simulink model "pry_grasp_source"  (R2018b)
settings: Solver=FixedStepDiscrete  StartTime=0.0  StopTime=Inf  FixedStep=0.001  RelTol=1e-3
PostLoadFcn:
  | , if any(exist('dsrtsu_mdlpostloadfcn', 'file') ~= 0), dsrtsu_mdlpostloadfcn('Execute', bdroot); end,
undefined symbols (not defined in the file): b, Coulomb_friction, parallel_grasp, q1ini, q2ini, theta1, theta2, theta5, theta6, viscous_friction
libraries: simulink x26
(part 2 of 3)

== system pry_grasp_source/phase1/Enabled Subsystem7 ==
  enable : Inport
  angle_ref : Inport  Port=2
  angle : Inport  Port=3
  angle_vel : Inport  Port=4
  phase_time : Inport  Port=5
  end_time : Inport  Port=6
  Subsystem : Subsystem
  Triggered Subsystem : Subsystem  TreatAsAtomicUnit=on
  torque_out : Outport  OutputWhenDisabled=reset  InitialOutput=0
  wires:
  angle/1 -> Subsystem/6(current_angle), Triggered Subsystem/1(angle_In1)
  angle_ref/1 -> Triggered Subsystem/2(angle_ref_In2)
  end_time/1 -> Triggered Subsystem/3(end_time_In3)
  Triggered Subsystem/1(angle_Out1) -> Subsystem/1(initial_angle)
  Triggered Subsystem/2(angle_ref_Out2) -> Subsystem/2(end_angle)
  Triggered Subsystem/3(end_time_Out3) -> Subsystem/3(end_time)
  phase_time/1 -> Subsystem/4(time)
  angle_vel/1 -> Subsystem/5(angular_vel)
  Subsystem/1(torque_out) -> torque_out/1
  enable/1 -> Triggered Subsystem/Trigger, Subsystem/Enable

== system pry_grasp_source/phase1/Triggered Subsystem ==
  note: arm move downward
  In1 : Inport
  Trigger : TriggerPort  VariantControl=(inherit)
  Constant : Constant  Value=[0 1]
  Constant1 : Constant  Value=1.5
  Data Store Read : DataStoreRead  Priority=3  DataStoreName=phase_num
  Data Store Read4 : DataStoreRead  Priority=3  DataStoreName=UR_V
  Data Store Write : DataStoreWrite  DataStoreName=phase_num
  Data Store Write4 : DataStoreWrite  DataStoreName=UR_V
  Sum : Sum  Inputs=|++
  Sum1 : Sum  Inputs=|++
  Out1 : Outport
  wires:
  Data Store Read/1 -> Sum/1
  Sum/1 -> Data Store Write/1
  Constant/1 -> Sum/2
  Constant1/1 -> Sum1/2
  Sum1/1 -> Data Store Write4/1
  Data Store Read4/1 -> Sum1/1
  In1/1 -> Out1/1

== system pry_grasp_source/phase1/Triggered Subsystem1 ==
  In1 : Inport
  Trigger : TriggerPort  VariantControl=(inherit)
  Out1 : Outport  InitialOutput=0
  wires:
  In1/1 -> Out1/1

== system pry_grasp_source/phase1-1/Enabled Subsystem ==
  phase_start_time : Inport
  current_time : Inport  Port=2
  phase_end_time : Inport  Port=3
  Enable : EnablePort
  Relational Operator : RelationalOperator  OutDataTypeStr=boolean  RndMeth=Nearest
  Sum : Sum  Inputs=|-+
  phase_time : Outport  OutputWhenDisabled=reset  InitialOutput=0
  phase_end_signal : Outport  Port=2  OutputWhenDisabled=reset  InitialOutput=0
  wires:
  phase_start_time/1 -> Sum/1
  current_time/1 -> Sum/2
  Sum/1 -> phase_time/1, Relational Operator/1
  Relational Operator/1 -> phase_end_signal/1
  phase_end_time/1 -> Relational Operator/2

== system pry_grasp_source/phase1-1/Enabled Subsystem7 ==
  enable : Inport
  angle_ref : Inport  Port=2
  angle : Inport  Port=3
  angle_vel : Inport  Port=4
  Subsystem : Subsystem
  torque_out : Outport  OutputWhenDisabled=reset  InitialOutput=0
  wires:
  angle/1 -> Subsystem/3(current_angle)
  angle_ref/1 -> Subsystem/1(ref_angle)
  angle_vel/1 -> Subsystem/2(angular_vel)
  Subsystem/1(torque_out) -> torque_out/1
  enable/1 -> Subsystem/Enable

== system pry_grasp_source/phase1-1/Triggered Subsystem ==
  Trigger : TriggerPort  VariantControl=(inherit)
  Constant : Constant  Value=[0 1]
  Data Store Read : DataStoreRead  Priority=3  DataStoreName=phase_num
  Data Store Write : DataStoreWrite  DataStoreName=phase_num
  Sum : Sum  Inputs=|++
  wires:
  Data Store Read/1 -> Sum/1
  Sum/1 -> Data Store Write/1
  Constant/1 -> Sum/2

== system pry_grasp_source/phase1-1/Triggered Subsystem1 ==
  In1 : Inport
  Trigger : TriggerPort  VariantControl=(inherit)
  Out1 : Outport  InitialOutput=0
  wires:
  In1/1 -> Out1/1

== system pry_grasp_source/phase10/Enabled Subsystem1 ==
  In1 : Inport
  Enable : EnablePort
  Out1 : Outport  OutputWhenDisabled=reset  InitialOutput=0
  wires:
  In1/1 -> Out1/1

== system pry_grasp_source/phase10/Enabled Subsystem3 ==
  phase_start_time : Inport
  current_time : Inport  Port=2
  phase_end_time : Inport  Port=3
  Enable : EnablePort
  Relational Operator : RelationalOperator  OutDataTypeStr=boolean  RndMeth=Nearest
  Sum : Sum  Inputs=|-+
  phase_time : Outport  OutputWhenDisabled=reset  InitialOutput=0
  phase_end_signal : Outport  Port=2  OutputWhenDisabled=reset  InitialOutput=0
  wires:
  phase_start_time/1 -> Sum/1
  current_time/1 -> Sum/2
  Sum/1 -> phase_time/1, Relational Operator/1
  Relational Operator/1 -> phase_end_signal/1
  phase_end_time/1 -> Relational Operator/2

== system pry_grasp_source/phase10/Enabled Subsystem4 ==
  enable : Inport
  angle6 : Inport  Port=2
  angle5 : Inport  Port=3
  angular5_vel : Inport  Port=4
  angular6_vel : Inport  Port=5
  angle1 : Inport  Port=6
  angle2 : Inport  Port=7
  angular1_vel : Inport  Port=8
  angular2_vel : Inport  Port=9
  vel_x1 : Inport  Port=10
  Subsystem1 : Subsystem
  torque_out : Outport  OutputWhenDisabled=reset  InitialOutput=0
  wires:
  enable/1 -> Subsystem1/Enable
  Subsystem1/1(torque) -> torque_out/1
  angle5/1 -> Subsystem1/2(angle5)
  angle6/1 -> Subsystem1/1(angle6)
  angular5_vel/1 -> Subsystem1/3(angular5_vel)
  angular6_vel/1 -> Subsystem1/4(angular6_vel)
  angle1/1 -> Subsystem1/6(angle1)
  angle2/1 -> Subsystem1/5("angle2 ")
  angular1_vel/1 -> Subsystem1/7(angular1_vel)
  angular2_vel/1 -> Subsystem1/8(angular2_vel)
  vel_x1/1 -> Subsystem1/9(vel_x1)

== system pry_grasp_source/phase10/Triggered Subsystem1 ==
  Trigger : TriggerPort  VariantControl=(inherit)
  Constant : Constant  Value=[0 1]
  Data Store Read : DataStoreRead  Priority=3  DataStoreName=phase_num
  Data Store Write : DataStoreWrite  DataStoreName=phase_num
  Sum : Sum  Inputs=|++
  wires:
  Data Store Read/1 -> Sum/1
  Sum/1 -> Data Store Write/1
  Constant/1 -> Sum/2

== system pry_grasp_source/phase10/Triggered Subsystem4 ==
  Trigger : TriggerPort  VariantControl=(inherit)
  Constant : Constant  Value=[0 1]
  Data Store Read : DataStoreRead  Priority=3  DataStoreName=phase_num
  Data Store Write : DataStoreWrite  DataStoreName=phase_num
  Sum : Sum  Inputs=|++
  wires:
  Data Store Read/1 -> Sum/1
  Sum/1 -> Data Store Write/1
  Constant/1 -> Sum/2

== system pry_grasp_source/phase10/Triggered Subsystem5 ==
  In1 : Inport
  Trigger : TriggerPort  VariantControl=(inherit)
  Out1 : Outport  InitialOutput=0
  wires:
  In1/1 -> Out1/1

== system pry_grasp_source/phase11/Enabled Subsystem2 ==
  In1 : Inport
  Enable : EnablePort
  Out1 : Outport  OutputWhenDisabled=reset  InitialOutput=0
  wires:
  In1/1 -> Out1/1

== system pry_grasp_source/phase11/Enabled Subsystem3 ==
  phase_start_time : Inport
  current_time : Inport  Port=2
  phase_end_time : Inport  Port=3
  Enable : EnablePort
  Relational Operator : RelationalOperator  OutDataTypeStr=boolean  RndMeth=Nearest
  Sum : Sum  Inputs=|-+
  phase_time : Outport  OutputWhenDisabled=reset  InitialOutput=0
  phase_end_signal : Outport  Port=2  OutputWhenDisabled=reset  InitialOutput=0
  wires:
  phase_start_time/1 -> Sum/1
  current_time/1 -> Sum/2
  Sum/1 -> phase_time/1, Relational Operator/1
  Relational Operator/1 -> phase_end_signal/1
  phase_end_time/1 -> Relational Operator/2

== system pry_grasp_source/phase11/Enabled Subsystem4 ==
  enable : Inport
  angular5_in1 : Inport  Port=2
  angle2 : Inport  Port=3
  angle1 : Inport  Port=4
  angle6 : Inport  Port=5
  angle5 : Inport  Port=6
  Subsystem1 : Subsystem
  torque_out : Outport  OutputWhenDisabled=reset  InitialOutput=0
  wires:
  enable/1 -> Subsystem1/Enable
  Subsystem1/1(torque) -> torque_out/1
  angular5_in1/1 -> ?
  angle1/1 -> Subsystem1/2(angle1)
  angle2/1 -> Subsystem1/1("angle2 ")
  angle5/1 -> Subsystem1/4(angle5)
  angle6/1 -> Subsystem1/3(angle6)

== system pry_grasp_source/phase11/Triggered Subsystem3 ==
  In1 : Inport
  Trigger : TriggerPort  VariantControl=(inherit)
  Constant : Constant  Value=[0 1]
  Data Store Read : DataStoreRead  Priority=3  DataStoreName=phase_num
  Data Store Write : DataStoreWrite  DataStoreName=phase_num
  Sum : Sum  Inputs=|++
  Out1 : Outport
  wires:
  Data Store Read/1 -> Sum/1
  Sum/1 -> Data Store Write/1
  Constant/1 -> Sum/2
  In1/1 -> Out1/1

== system pry_grasp_source/phase11/Triggered Subsystem4 ==
  Trigger : TriggerPort  VariantControl=(inherit)
  Constant : Constant  Value=[0 1]
  Data Store Read : DataStoreRead  Priority=3  DataStoreName=phase_num
  Data Store Write : DataStoreWrite  DataStoreName=phase_num
  Sum : Sum  Inputs=|++
  wires:
  Data Store Read/1 -> Sum/1
  Sum/1 -> Data Store Write/1
  Constant/1 -> Sum/2

== system pry_grasp_source/phase11/Triggered Subsystem5 ==
  In1 : Inport
  Trigger : TriggerPort  VariantControl=(inherit)
  Out1 : Outport  InitialOutput=0
  wires:
  In1/1 -> Out1/1

== system pry_grasp_source/phase2/Enabled Subsystem ==
  phase_start_time : Inport
  current_time : Inport  Port=2
  phase_end_time : Inport  Port=3
  Enable : EnablePort
  Relational Operator : RelationalOperator  OutDataTypeStr=boolean  RndMeth=Nearest
  Sum : Sum  Inputs=|-+
  phase_time : Outport  OutputWhenDisabled=reset  InitialOutput=0
  phase_end_signal : Outport  Port=2  OutputWhenDisabled=reset  InitialOutput=0
  wires:
  phase_start_time/1 -> Sum/1
  current_time/1 -> Sum/2
  Sum/1 -> phase_time/1, Relational Operator/1
  Relational Operator/1 -> phase_end_signal/1
  phase_end_time/1 -> Relational Operator/2

== system pry_grasp_source/phase2/Enabled Subsystem7 ==
  enable : Inport
  ref_angle : Inport  Port=2
  angle : Inport  Port=3
  angle_vel : Inport  Port=4
  Subsystem : Subsystem
  torque_out : Outport  OutputWhenDisabled=reset  InitialOutput=0
  wires:
  angle/1 -> Subsystem/3(current_angle)
  angle_vel/1 -> Subsystem/2(angular_vel)
  Subsystem/1(torque_out) -> torque_out/1
  enable/1 -> Subsystem/Enable
  ref_angle/1 -> Subsystem/1(ref_angle)

== system pry_grasp_source/phase2/Triggered Subsystem ==
  In1 : Inport
  Trigger : TriggerPort  VariantControl=(inherit)
  Constant : Constant  Value=[0 1]
  Constant1 : Constant
  Data Store Read : DataStoreRead  Priority=3  DataStoreName=phase_num
  Data Store Read4 : DataStoreRead  Priority=3  DataStoreName=UR_V
  Data Store Write : DataStoreWrite  DataStoreName=phase_num
  Data Store Write4 : DataStoreWrite  DataStoreName=UR_V
  Sum : Sum  Inputs=|++
  Sum1 : Sum  Inputs=|++
  Out1 : Outport
  wires:
  Data Store Read/1 -> Sum/1
  Sum/1 -> Data Store Write/1
  Constant/1 -> Sum/2
  In1/1 -> Out1/1
  Constant1/1 -> Sum1/2
  Data Store Read4/1 -> Sum1/1
  Sum1/1 -> Data Store Write4/1

== system pry_grasp_source/phase2/Triggered Subsystem1 ==
  In1 : Inport
  Trigger : TriggerPort  VariantControl=(inherit)
  Out1 : Outport  InitialOutput=0
  wires:
  In1/1 -> Out1/1

== system pry_grasp_source/phase6.1/Enabled Subsystem ==
  phase_start_time : Inport
  current_time : Inport  Port=2
  phase_end_time : Inport  Port=3
  Enable : EnablePort
  Relational Operator : RelationalOperator  OutDataTypeStr=boolean  RndMeth=Nearest
  Sum : Sum  Inputs=|-+
  phase_time : Outport  OutputWhenDisabled=reset  InitialOutput=0
  phase_end_signal : Outport  Port=2  OutputWhenDisabled=reset  InitialOutput=0
  wires:
  phase_start_time/1 -> Sum/1
  current_time/1 -> Sum/2
  Sum/1 -> phase_time/1, Relational Operator/1
  Relational Operator/1 -> phase_end_signal/1
  phase_end_time/1 -> Relational Operator/2

== system pry_grasp_source/phase6.1/Enabled Subsystem2 ==
  In1 : Inport
  Enable : EnablePort
  Out1 : Outport  OutputWhenDisabled=reset  InitialOutput=0
  wires:
  In1/1 -> Out1/1

== system pry_grasp_source/phase6.1/Enabled Subsystem7 ==
  enable : Inport
  angle_ref : Inport  Port=2
  angle : Inport  Port=3
  angle_vel : Inport  Port=4
  phase_time : Inport  Port=5
  end_time : Inport  Port=6
  Subsystem : Subsystem
  Triggered Subsystem : Subsystem  TreatAsAtomicUnit=on
  tau_out : Outport
  wires:
  angle/1 -> Subsystem/6(current_angle), Triggered Subsystem/1(angle_In1)
  angle_ref/1 -> Triggered Subsystem/2(angle_ref_In2)
  end_time/1 -> Triggered Subsystem/3(end_time_In3)
  Triggered Subsystem/1(angle_Out1) -> Subsystem/1(initial_angle)
  Triggered Subsystem/2(angle_ref_Out2) -> Subsystem/2(end_angle)
  Triggered Subsystem/3(end_time_Out3) -> Subsystem/3(end_time)
  phase_time/1 -> Subsystem/4(time)
  angle_vel/1 -> Subsystem/5(angular_vel)
  Subsystem/1(tau_out) -> tau_out/1
  enable/1 -> Triggered Subsystem/Trigger, Subsystem/Enable

== system pry_grasp_source/phase6.1/Triggered Subsystem ==
  In1 : Inport
  Trigger : TriggerPort  VariantControl=(inherit)
  Constant : Constant  Value=[0 0.1]
  Data Store Read : DataStoreRead  Priority=3  DataStoreName=phase_num
  Data Store Write : DataStoreWrite  DataStoreName=phase_num
  Sum : Sum  Inputs=|++
  Out1 : Outport
  wires:
  Data Store Read/1 -> Sum/1
  Sum/1 -> Data Store Write/1
  Constant/1 -> Sum/2
  In1/1 -> Out1/1

== system pry_grasp_source/phase6.1/Triggered Subsystem1 ==
  In1 : Inport
  Trigger : TriggerPort  VariantControl=(inherit)
  Out1 : Outport  InitialOutput=0
  wires:
  In1/1 -> Out1/1

== system pry_grasp_source/phase6.1/Triggered Subsystem3 ==
  Trigger : TriggerPort  VariantControl=(inherit)
  Constant : Constant  Value=[0 1]
  Data Store Read : DataStoreRead  Priority=3  DataStoreName=phase_num
  Data Store Write : DataStoreWrite  DataStoreName=phase_num
  Sum : Sum  Inputs=|++
  wires:
  Data Store Read/1 -> Sum/1
  Sum/1 -> Data Store Write/1
  Constant/1 -> Sum/2

== system pry_grasp_source/phase700/Enabled Subsystem ==
  phase_start_time : Inport
  current_time : Inport  Port=2
  phase_end_time : Inport  Port=3
  Enable : EnablePort
  Relational Operator : RelationalOperator  OutDataTypeStr=boolean  RndMeth=Nearest
  Sum : Sum  Inputs=|-+
  phase_time : Outport  OutputWhenDisabled=reset  InitialOutput=0
  phase_end_signal : Outport  Port=2  OutputWhenDisabled=reset  InitialOutput=0
  wires:
  phase_start_time/1 -> Sum/1
  current_time/1 -> Sum/2
  Sum/1 -> phase_time/1, Relational Operator/1
  Relational Operator/1 -> phase_end_signal/1
  phase_end_time/1 -> Relational Operator/2

== system pry_grasp_source/phase700/Enabled Subsystem2 ==
  In1 : Inport
  Enable : EnablePort
  Out1 : Outport  OutputWhenDisabled=reset  InitialOutput=0
  wires:
  In1/1 -> Out1/1

== system pry_grasp_source/phase700/Enabled Subsystem7 ==
  enable : Inport
  angle_ref : Inport  Port=2
  angle : Inport  Port=3
  angle_vel : Inport  Port=4
  phase_time : Inport  Port=5
  end_time : Inport  Port=6
  Subsystem : Subsystem
  Triggered Subsystem : Subsystem  TreatAsAtomicUnit=on
  torque_out : Outport  OutputWhenDisabled=reset  InitialOutput=0
  wires:
  angle/1 -> Subsystem/6(current_angle), Triggered Subsystem/1(angle_In1)
  angle_ref/1 -> Triggered Subsystem/2(angle_ref_In2)
  end_time/1 -> Triggered Subsystem/3(end_time_In3)
  Triggered Subsystem/1(angle_Out1) -> Subsystem/1(initial_angle)
  Triggered Subsystem/2(angle_ref_Out2) -> Subsystem/2(end_angle)
  Triggered Subsystem/3(end_time_Out3) -> Subsystem/3(end_time)
  phase_time/1 -> Subsystem/4(time)
  angle_vel/1 -> Subsystem/5(angular_vel)
  Subsystem/1(torque_out) -> torque_out/1
  enable/1 -> Triggered Subsystem/Trigger, Subsystem/Enable

== system pry_grasp_source/phase700/Subsystem1 ==
  note: 判断物体是否接触到左侧手指
  initial_angle2 : Inport
  Enable : EnablePort
  Delay : Delay  DelayLength=5  InitialCondition=0
  Sum : Sum  Inputs=|+-
  Triggered Subsystem3 : Subsystem  TreatAsAtomicUnit=on
  angle2_the : simulink/Logic and Bit Operations/Compare To Constant  relop=<=  const=-0.023  OutDataTypeStr=uint8
  jump : Gain
  wires:
  initial_angle2/1 -> Delay/1, Sum/1
  Delay/1 -> Sum/2
  Sum/1 -> angle2_the/1
  angle2_the/1 -> jump/1, Triggered Subsystem3/Trigger

== system pry_grasp_source/phase700/Triggered Subsystem ==
  note: arm停止运动
  In1 : Inport
  Trigger : TriggerPort  VariantControl=(inherit)
  Constant : Constant  Value=[0 1]
  Constant1 : Constant  Value=2
  Data Store Read : DataStoreRead  Priority=3  DataStoreName=phase_num
  Data Store Read4 : DataStoreRead  Priority=3  DataStoreName=UR_V
  Data Store Write : DataStoreWrite  DataStoreName=phase_num
  Data Store Write4 : DataStoreWrite  DataStoreName=UR_V
  Sum : Sum  Inputs=|++
  Sum1 : Sum  Inputs=|++
  Out1 : Outport
  wires:
  Data Store Read/1 -> Sum/1
  Sum/1 -> Data Store Write/1
  Constant/1 -> Sum/2
  In1/1 -> Out1/1
  Sum1/1 -> Data Store Write4/1
  Constant1/1 -> Sum1/2
  Data Store Read4/1 -> Sum1/1

== system pry_grasp_source/phase700/Triggered Subsystem1 ==
  In1 : Inport
  Trigger : TriggerPort  VariantControl=(inherit)
  Out1 : Outport  InitialOutput=0
  wires:
  In1/1 -> Out1/1

== system pry_grasp_source/phase700/Triggered Subsystem3 ==
  In1 : Inport
  Trigger : TriggerPort  VariantControl=(inherit)
  Constant : Constant  Value=[0 1]
  Data Store Read : DataStoreRead  Priority=3  DataStoreName=phase_num
  Data Store Write : DataStoreWrite  DataStoreName=phase_num
  Sum : Sum  Inputs=|++
  Out1 : Outport
  wires:
  Data Store Read/1 -> Sum/1
  Sum/1 -> Data Store Write/1
  Constant/1 -> Sum/2
  In1/1 -> Out1/1

== system pry_grasp_source/phase90/Enabled Subsystem2 ==
  In1 : Inport
  Enable : EnablePort
  Out1 : Outport  OutputWhenDisabled=reset  InitialOutput=0
  wires:
  In1/1 -> Out1/1

== system pry_grasp_source/phase90/Enabled Subsystem3 ==
  phase_start_time : Inport
  current_time : Inport  Port=2
  phase_end_time : Inport  Port=3
  Enable : EnablePort
  Relational Operator : RelationalOperator  OutDataTypeStr=boolean  RndMeth=Nearest
  Sum : Sum  Inputs=|-+
  phase_time : Outport  OutputWhenDisabled=reset  InitialOutput=0
  phase_end_signal : Outport  Port=2  OutputWhenDisabled=reset  InitialOutput=0
  wires:
  phase_start_time/1 -> Sum/1
  current_time/1 -> Sum/2
  Sum/1 -> phase_time/1, Relational Operator/1
  Relational Operator/1 -> phase_end_signal/1
  phase_end_time/1 -> Relational Operator/2

== system pry_grasp_source/phase90/Enabled Subsystem4 ==
  note: 关节5的角度值
  phase time : Inport
  angular5_vel : Inport  Port=2
  angle5_ref : Inport  Port=3
  end_time : Inport  Port=4
  enable : Inport  Port=5
  angle2 : Inport  Port=6
  angle5_in : Inport  Port=7
  angle1 : Inport  Port=8
  Subsystem1 : Subsystem
  Triggered Subsystem : Subsystem  TreatAsAtomicUnit=on
  torque_out : Outport  OutputWhenDisabled=reset  InitialOutput=0
  wires:
  angle5_ref/1 -> Triggered Subsystem/2(angle5_ref)
  Triggered Subsystem/2(angle5_ref_Out) -> Subsystem1/2(end_angle5)
  end_time/1 -> Triggered Subsystem/3(end_time)
  enable/1 -> Triggered Subsystem/Trigger, Subsystem1/Enable
  Triggered Subsystem/1(angle5_Out) -> Subsystem1/1(initial_angle5)
  Triggered Subsystem/3(end_time_Out) -> Subsystem1/3(end_time)
  phase time/1 -> Subsystem1/4(time)
  angular5_vel/1 -> Subsystem1/5(angular5_vel)
  angle5_in/1 -> Subsystem1/6(current_angle5), Triggered Subsystem/1(angle5_In)
  angle2/1 -> Subsystem1/7("angle2 ")
  Subsystem1/1(torque) -> torque_out/1
  angle1/1 -> Subsystem1/8(angle1)

== system pry_grasp_source/phase90/Triggered Subsystem3 ==
  Trigger : TriggerPort  VariantControl=(inherit)
  Constant : Constant  Value=[0 1]
  Data Store Read : DataStoreRead  Priority=3  DataStoreName=phase_num
  Data Store Write : DataStoreWrite  DataStoreName=phase_num
  Sum : Sum  Inputs=|++
  wires:
  Data Store Read/1 -> Sum/1
  Sum/1 -> Data Store Write/1
  Constant/1 -> Sum/2

== system pry_grasp_source/phase90/Triggered Subsystem4 ==
  Trigger : TriggerPort  VariantControl=(inherit)
  Constant : Constant  Value=[0 1]
  Data Store Read : DataStoreRead  Priority=3  DataStoreName=phase_num
  Data Store Write : DataStoreWrite  DataStoreName=phase_num
  Sum : Sum  Inputs=|++
  wires:
  Data Store Read/1 -> Sum/1
  Sum/1 -> Data Store Write/1
  Constant/1 -> Sum/2

== system pry_grasp_source/phase90/Triggered Subsystem5 ==
  In1 : Inport
  Trigger : TriggerPort  VariantControl=(inherit)
  Out1 : Outport  InitialOutput=0
  wires:
  In1/1 -> Out1/1

== system pry_grasp_source/prying motion/Enabled Subsystem1 ==
  In1 : Inport
  Enable : EnablePort
  Out1 : Outport  OutputWhenDisabled=reset  InitialOutput=0
  wires:
  In1/1 -> Out1/1

== system pry_grasp_source/prying motion/Enabled Subsystem3 ==
  phase_start_time : Inport
  current_time : Inport  Port=2
  phase_end_time : Inport  Port=3
  Enable : EnablePort
  Relational Operator : RelationalOperator  OutDataTypeStr=boolean  RndMeth=Nearest
  Sum : Sum  Inputs=|-+
  phase_time : Outport  OutputWhenDisabled=reset  InitialOutput=0
  phase_end_signal : Outport  Port=2  OutputWhenDisabled=reset  InitialOutput=0
  wires:
  phase_start_time/1 -> Sum/1
  current_time/1 -> Sum/2
  Sum/1 -> phase_time/1, Relational Operator/1
  Relational Operator/1 -> phase_end_signal/1
  phase_end_time/1 -> Relational Operator/2

== system pry_grasp_source/prying motion/Enabled Subsystem4 ==
  enable : Inport
  pry force : Inport  Port=2
  angle2 : Inport  Port=3
  angle1 : Inport  Port=4
  angle6 : Inport  Port=5
  angle5 : Inport  Port=6
  Subsystem1 : Subsystem
  torque_out : Outport  OutputWhenDisabled=reset  InitialOutput=0
  wires:
  enable/1 -> Subsystem1/Enable
  Subsystem1/1(torque) -> torque_out/1
  angle1/1 -> Subsystem1/3(angle1)
  angle2/1 -> Subsystem1/2("angle2 ")
  angle5/1 -> Subsystem1/5(angle5)
  angle6/1 -> Subsystem1/4(angle6)
  pry force/1 -> Subsystem1/1(pry force)

== system pry_grasp_source/prying motion/Enabled Subsystem6 ==
  In1 : Inport
  Enable : EnablePort
  Out1 : Outport  OutputWhenDisabled=reset  InitialOutput=0
  wires:
  In1/1 -> Out1/1

== system pry_grasp_source/prying motion/Enabled Subsystem7 ==
  time : Inport
  k : Inport  Port=2
  F_end : Inport  Port=3
  Enable : EnablePort
  MATLAB Function : MATLAB Function  TreatAsAtomicUnit=on
  q7 q8 : Constant  Value=[0 0]
  Out1 : Outport
  wires:
  q7 q8/1 -> ?
  time/1 -> MATLAB Function/1(time)
  k/1 -> MATLAB Function/2(k)
  MATLAB Function/1(F_o) -> Out1/1
  F_end/1 -> MATLAB Function/3(F_end)

== system pry_grasp_source/prying motion/Triggered Subsystem1 ==
  In1 : Inport
  Trigger : TriggerPort  VariantControl=(inherit)
  Constant : Constant  Value=[0 1]
  Data Store Read : DataStoreRead  Priority=3  DataStoreName=phase_num
  Data Store Read2 : DataStoreRead  DataStoreName=stop_force
  Data Store Write : DataStoreWrite  DataStoreName=phase_num
  Sum : Sum  Inputs=|++
  detected force : DataStoreWrite  DataStoreName=initial_force
  Out1 : Outport  OutputWhenDisabled=reset  InitialOutput=0
  wires:
  Data Store Read/1 -> Sum/1
  Sum/1 -> Data Store Write/1
  Constant/1 -> Sum/2
  In1/1 -> Out1/1
  Data Store Read2/1 -> detected force/1

== system pry_grasp_source/prying motion/Triggered Subsystem2 ==
  In1 : Inport
  Trigger : TriggerPort  VariantControl=(inherit)
  Constant : Constant  Value=[0 3]
  Data Store Read : DataStoreRead  Priority=3  DataStoreName=phase_num
  Data Store Read2 : DataStoreRead  DataStoreName=stop_force
  Data Store Write : DataStoreWrite  DataStoreName=phase_num
  Sum : Sum  Inputs=|++
  detected force : DataStoreWrite  DataStoreName=initial_force
  Out1 : Outport
  wires:
  Data Store Read/1 -> Sum/1
  Sum/1 -> Data Store Write/1
  Constant/1 -> Sum/2
  In1/1 -> Out1/1
  Data Store Read2/1 -> detected force/1

== system pry_grasp_source/prying motion/Triggered Subsystem4 ==
  Trigger : TriggerPort  VariantControl=(inherit)
  Constant : Constant  Value=[0 1]
  Data Store Read : DataStoreRead  Priority=3  DataStoreName=phase_num
  Data Store Write : DataStoreWrite  DataStoreName=phase_num
  Sum : Sum  Inputs=|++
  wires:
  Data Store Read/1 -> Sum/1
  Sum/1 -> Data Store Write/1
  Constant/1 -> Sum/2

== system pry_grasp_source/prying motion/Triggered Subsystem5 ==
  In1 : Inport
  Trigger : TriggerPort  VariantControl=(inherit)
  Out1 : Outport  InitialOutput=0
  wires:
  In1/1 -> Out1/1

== system pry_grasp_source/pusher drops to detect the table surface/Enabled Subsystem3 ==
  phase_start_time : Inport
  current_time : Inport  Port=2
  phase_end_time : Inport  Port=3
  Enable : EnablePort
  Relational Operator : RelationalOperator  OutDataTypeStr=boolean  RndMeth=Nearest
  Sum : Sum  Inputs=|-+
  phase_time : Outport  OutputWhenDisabled=reset  InitialOutput=0
  phase_end_signal : Outport  Port=2  OutputWhenDisabled=reset  InitialOutput=0
  wires:
  phase_start_time/1 -> Sum/1
  current_time/1 -> Sum/2
  Sum/1 -> phase_time/1, Relational Operator/1
  Relational Operator/1 -> phase_end_signal/1
  phase_end_time/1 -> Relational Operator/2

== system pry_grasp_source/pusher drops to detect the table surface/Triggered Subsystem4 ==
  In1 : Inport
  Trigger : TriggerPort  VariantControl=(inherit)
  Constant : Constant  Value=[0 1]
  Data Store Read : DataStoreRead  Priority=3  DataStoreName=phase_num
  Data Store Write : DataStoreWrite  DataStoreName=phase_num
  Sum : Sum  Inputs=|++
  angle_end : Outport
  wires:
  Data Store Read/1 -> Sum/1
  Sum/1 -> Data Store Write/1
  Constant/1 -> Sum/2
  In1/1 -> angle_end/1

== system pry_grasp_source/pusher drops to detect the table surface/Triggered Subsystem5 ==
  In1 : Inport
  Trigger : TriggerPort  VariantControl=(inherit)
  Out1 : Outport  InitialOutput=0
  wires:
  In1/1 -> Out1/1

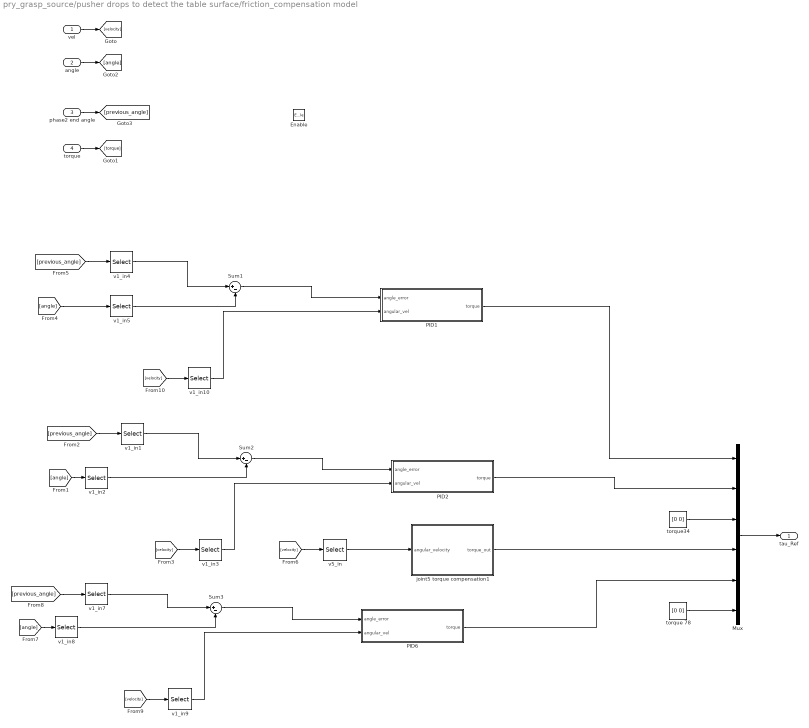
== system pry_grasp_source/pusher drops to detect the table surface/friction_compensation model ==
  vel : Inport
  angle : Inport  Port=2
  phase2 end angle : Inport  Port=3
  torque : Inport  Port=4
  Enable : EnablePort
  Mux : Mux  Inputs=6
  PID1 : Subsystem
  PID2 : Subsystem
  PID6 : Subsystem
  Sum1 : Sum  Inputs=|+-
  Sum2 : Sum  Inputs=|+-
  Sum3 : Sum  Inputs=|+-
  joint5 torque compensation1 : Subsystem
  torque 78 : Constant  Value=[0 0]
  torque34 : Constant  Value=[0 0]
  v1_in1 : Selector  InputPortWidth=8  IndexOptions=Index vector (dialog)  Indices=2  OutputSizes=1
  v1_in10 : Selector  InputPortWidth=8  IndexOptions=Index vector (dialog)  Indices=1  OutputSizes=1
  v1_in2 : Selector  InputPortWidth=8  IndexOptions=Index vector (dialog)  Indices=2  OutputSizes=1
  v1_in3 : Selector  InputPortWidth=8  IndexOptions=Index vector (dialog)  Indices=2  OutputSizes=1
  v1_in4 : Selector  InputPortWidth=8  IndexOptions=Index vector (dialog)  Indices=1  OutputSizes=1
  v1_in5 : Selector  InputPortWidth=8  IndexOptions=Index vector (dialog)  Indices=1  OutputSizes=1
  v1_in7 : Selector  InputPortWidth=8  IndexOptions=Index vector (dialog)  Indices=6  OutputSizes=1
  v1_in8 : Selector  InputPortWidth=8  IndexOptions=Index vector (dialog)  Indices=6  OutputSizes=1
  v1_in9 : Selector  InputPortWidth=8  IndexOptions=Index vector (dialog)  Indices=6  OutputSizes=1
  v5_in : Selector  InputPortWidth=8  IndexOptions=Index vector (dialog)  Indices=5  OutputSizes=1
  tau_Ref : Outport  InitialOutput=[0 0 0 0 0 0 0 0]
  wires:
  torque 78/1 -> Mux/6
  PID1/1(torque) -> Mux/1
  Mux/1 -> tau_Ref/1
  torque34/1 -> Mux/3
  PID6/1(torque) -> Mux/5
  vel/1 -> [velocity]
  torque/1 -> [torque]
  angle/1 -> [angle]
  phase2 end angle/1 -> [previous_angle]
  [previous_angle] -> v1_in1/1
  v1_in1/1 -> Sum2/1
  [angle] -> v1_in2/1
  v1_in2/1 -> Sum2/2
  Sum2/1 -> PID2/1(angle_error)
  [velocity] -> v1_in3/1
  v1_in3/1 -> PID2/2(angular_vel)
  PID2/1(torque) -> Mux/2
  [velocity] -> v5_in/1
  v5_in/1 -> joint5 torque compensation1/1(angular_velocity)
  v1_in7/1 -> Sum3/1
  [previous_angle] -> v1_in7/1
  [velocity] -> v1_in9/1
  Sum3/1 -> PID6/1(angle_error)
  v1_in8/1 -> Sum3/2
  [angle] -> v1_in8/1
  v1_in9/1 -> PID6/2(angular_vel)
  v1_in4/1 -> Sum1/1
  [angle] -> v1_in5/1
  Sum1/1 -> PID1/1(angle_error)
  v1_in5/1 -> Sum1/2
  [velocity] -> v1_in10/1
  [previous_angle] -> v1_in4/1
  v1_in10/1 -> PID1/2(angular_vel)
  joint5 torque compensation1/1(torque_out) -> Mux/4

== system pry_grasp_source/pusher pushes object/Enabled Subsystem3 ==
  phase_start_time : Inport
  current_time : Inport  Port=2
  phase_end_time : Inport  Port=3
  Enable : EnablePort
  Relational Operator : RelationalOperator  OutDataTypeStr=boolean  RndMeth=Nearest
  Sum : Sum  Inputs=|-+
  phase_time : Outport  OutputWhenDisabled=reset  InitialOutput=0
  phase_end_signal : Outport  Port=2  OutputWhenDisabled=reset  InitialOutput=0
  wires:
  phase_start_time/1 -> Sum/1
  current_time/1 -> Sum/2
  Sum/1 -> phase_time/1, Relational Operator/1
  Relational Operator/1 -> phase_end_signal/1
  phase_end_time/1 -> Relational Operator/2

== system pry_grasp_source/pusher pushes object/Enabled Subsystem4 ==
  note: desired y
  note: desired x
  phase time : Inport
  "angle2 " : Inport  Port=2
  angle1 : Inport  Port=3
  Constant2 : Constant  Value=0
  Fx_1_finger1 : Constant  Value=0
  Fy_1_finger1 : Constant  Value=0.1
  Gain : Gain  Gain=b
  MATLAB Function1 : MATLAB Function  TreatAsAtomicUnit=on
  MATLAB Function3 : MATLAB Function  TreatAsAtomicUnit=on
  MATLAB Function4 : MATLAB Function  TreatAsAtomicUnit=on
  Mux{,1..3} (4 alike) : Mux  Inputs=2
  Mux4 : Mux
  Sum : Sum  Inputs=|+-
  Sum1 : Sum  Inputs=|+-
  Sum2 : Sum  Inputs=|++
  Sum3 : Sum  Inputs=|++
  measured Fx : Constant  Value=0
  measured Fy : Constant  Value=0.1
  torque : Outport
  wires:
  [F_xd] -> Mux/1
  [F_yd] -> Mux/2
  measured Fx/1 -> Mux1/1
  measured Fy/1 -> Mux1/2
  Mux/1 -> Sum/1
  Mux1/1 -> Sum/2
  Sum/1 -> MATLAB Function3/1(F_e)
  Constant2/1 -> Mux2/2
  Mux2/1 -> Sum1/1
  Gain/1 -> Mux2/1
  Mux3/1 -> Sum1/2
  [P_y] -> Mux3/2
  Sum1/1 -> MATLAB Function4/1(P_e)
  [P_x] -> Mux3/1
  phase time/1 -> Gain/1
  Mux4/1 -> torque/1
  "angle2 "/1 -> MATLAB Function1/4(theta2_value)
  MATLAB Function1/2(tau2) -> Mux4/2
  Fy_1_finger1/1 -> MATLAB Function1/2(Fy_1)
  MATLAB Function1/1(tau1) -> Mux4/1
  Fx_1_finger1/1 -> MATLAB Function1/1(Fx_1)
  angle1/1 -> MATLAB Function1/3(theta1_value)
  MATLAB Function4/1(tau5s) -> Sum2/1
  MATLAB Function3/1(tau5f) -> Sum2/2
  MATLAB Function4/2(tau6s) -> Sum3/1
  MATLAB Function3/2(tau6f) -> Sum3/2
  Sum3/1 -> Mux4/4
  Sum2/1 -> Mux4/3

== system pry_grasp_source/pusher pushes object/Subsystem1 ==
  note: detect contact
  ve : Inport
  Enable : EnablePort
  Abs : Abs
  Triggered Subsystem3 : Subsystem  TreatAsAtomicUnit=on
  angle2_the : simulink/Logic and Bit Operations/Compare To Constant  relop=<=  const=0.1  OutDataTypeStr=uint8
  wires:
  angle2_the/1 -> Triggered Subsystem3/Trigger
  ve/1 -> Abs/1
  Abs/1 -> angle2_the/1

== system pry_grasp_source/pusher pushes object/Triggered Subsystem4 ==
  Trigger : TriggerPort  VariantControl=(inherit)
  Constant : Constant  Value=[0 1]
  Data Store Read : DataStoreRead  Priority=3  DataStoreName=phase_num
  Data Store Write : DataStoreWrite  DataStoreName=phase_num
  Sum : Sum  Inputs=|++
  wires:
  Data Store Read/1 -> Sum/1
  Sum/1 -> Data Store Write/1
  Constant/1 -> Sum/2

== system pry_grasp_source/pusher pushes object/Triggered Subsystem5 ==
  In1 : Inport
  Trigger : TriggerPort  VariantControl=(inherit)
  Out1 : Outport  InitialOutput=0
  wires:
  In1/1 -> Out1/1

== system pry_grasp_source/return to initial angle/Enabled Subsystem ==
  phase_start_time : Inport
  current_time : Inport  Port=2
  phase_end_time : Inport  Port=3
  Enable : EnablePort
  Relational Operator : RelationalOperator  OutDataTypeStr=boolean  RndMeth=Nearest
  Sum : Sum  Inputs=|-+
  phase_time : Outport  OutputWhenDisabled=reset  InitialOutput=0
  phase_end_signal : Outport  Port=2  OutputWhenDisabled=reset  InitialOutput=0
  wires:
  phase_start_time/1 -> Sum/1
  current_time/1 -> Sum/2
  Sum/1 -> phase_time/1, Relational Operator/1
  Relational Operator/1 -> phase_end_signal/1
  phase_end_time/1 -> Relational Operator/2

== system pry_grasp_source/return to initial angle/Enabled Subsystem7 ==
  enable : Inport
  angle_ref : Inport  Port=2
  angle : Inport  Port=3
  angle_vel : Inport  Port=4
  phase_time : Inport  Port=5
  end_time : Inport  Port=6
  Subsystem : Subsystem
  Triggered Subsystem : Subsystem  TreatAsAtomicUnit=on
  torque_out : Outport  OutputWhenDisabled=reset  InitialOutput=0
  wires:
  angle/1 -> Subsystem/6(current_angle), Triggered Subsystem/1(angle_In1)
  angle_ref/1 -> Triggered Subsystem/2(angle_ref_In2)
  end_time/1 -> Triggered Subsystem/3(end_time_In3)
  Triggered Subsystem/1(angle_Out1) -> Subsystem/1(initial_angle)
  Triggered Subsystem/2(angle_ref_Out2) -> Subsystem/2(end_angle)
  Triggered Subsystem/3(end_time_Out3) -> Subsystem/3(end_time)
  phase_time/1 -> Subsystem/4(time)
  angle_vel/1 -> Subsystem/5(angular_vel)
  Subsystem/1(torque_out) -> torque_out/1
  enable/1 -> Triggered Subsystem/Trigger, Subsystem/Enable

== system pry_grasp_source/return to initial angle/Triggered Subsystem ==
  Trigger : TriggerPort  VariantControl=(inherit)
  Constant : Constant  Value=[0 -3]
  Data Store Read : DataStoreRead  Priority=3  DataStoreName=phase_num
  Data Store Write : DataStoreWrite  DataStoreName=phase_num
  Sum : Sum  Inputs=|++
  wires:
  Data Store Read/1 -> Sum/1
  Sum/1 -> Data Store Write/1
  Constant/1 -> Sum/2

== system pry_grasp_source/return to initial angle/Triggered Subsystem1 ==
  In1 : Inport
  Trigger : TriggerPort  VariantControl=(inherit)
  Out1 : Outport  InitialOutput=0
  wires:
  In1/1 -> Out1/1

== system pry_grasp_source/return to initial position/Enabled Subsystem ==
  phase_start_time : Inport
  current_time : Inport  Port=2
  phase_end_time : Inport  Port=3
  Enable : EnablePort
  Relational Operator : RelationalOperator  OutDataTypeStr=boolean  RndMeth=Nearest
  Sum : Sum  Inputs=|-+
  phase_time : Outport  OutputWhenDisabled=reset  InitialOutput=0
  phase_end_signal : Outport  Port=2  OutputWhenDisabled=reset  InitialOutput=0
  wires:
  phase_start_time/1 -> Sum/1
  current_time/1 -> Sum/2
  Sum/1 -> phase_time/1, Relational Operator/1
  Relational Operator/1 -> phase_end_signal/1
  phase_end_time/1 -> Relational Operator/2

== system pry_grasp_source/return to initial position/Enabled Subsystem7 ==
  enable : Inport
  angle_ref : Inport  Port=2
  angle : Inport  Port=3
  angle_vel : Inport  Port=4
  phase_time : Inport  Port=5
  end_time : Inport  Port=6
  Subsystem : Subsystem
  Triggered Subsystem : Subsystem  TreatAsAtomicUnit=on
  tau_out : Outport
  wires:
  angle/1 -> Subsystem/6(current_angle), Triggered Subsystem/1(angle_In1)
  angle_ref/1 -> Triggered Subsystem/2(angle_ref_In2)
  end_time/1 -> Triggered Subsystem/3(end_time_In3)
  Triggered Subsystem/1(angle_Out1) -> Subsystem/1(initial_angle)
  Triggered Subsystem/2(angle_ref_Out2) -> Subsystem/2(end_angle)
  Triggered Subsystem/3(end_time_Out3) -> Subsystem/3(end_time)
  phase_time/1 -> Subsystem/4(time)
  angle_vel/1 -> Subsystem/5(angular_vel)
  Subsystem/1(tau_out) -> tau_out/1
  enable/1 -> Triggered Subsystem/Trigger, Subsystem/Enable

== system pry_grasp_source/return to initial position/Triggered Subsystem ==
  In1 : Inport
  Trigger : TriggerPort  VariantControl=(inherit)
  Constant : Constant  Value=[0 1]
  Data Store Read : DataStoreRead  Priority=3  DataStoreName=phase_num
  Data Store Write : DataStoreWrite  DataStoreName=phase_num
  Sum : Sum  Inputs=|++
  Out1 : Outport
  wires:
  Data Store Read/1 -> Sum/1
  Sum/1 -> Data Store Write/1
  Constant/1 -> Sum/2
  In1/1 -> Out1/1

== system pry_grasp_source/return to initial position/Triggered Subsystem1 ==
  In1 : Inport
  Trigger : TriggerPort  VariantControl=(inherit)
  Out1 : Outport  InitialOutput=0
  wires:
  In1/1 -> Out1/1

== system pry_grasp_source/tentatively push/Enabled Subsystem1 ==
  phase time : Inport
  angular_vel : Inport  Port=2
  angle_ref : Inport  Port=3
  end_time : Inport  Port=4
  enable : Inport  Port=5
  angle_in : Inport  Port=6
  Subsystem1 : Subsystem
  Triggered Subsystem : Subsystem  TreatAsAtomicUnit=on
  torque_out : Outport  OutputWhenDisabled=reset  InitialOutput=0
  wires:
  angle_ref/1 -> Triggered Subsystem/2(angle_ref)
  Triggered Subsystem/2(angle_ref_Out) -> Subsystem1/2(end_angle)
  end_time/1 -> Triggered Subsystem/3(end_time)
  enable/1 -> Triggered Subsystem/Trigger, Subsystem1/Enable
  Triggered Subsystem/3(end_time_Out) -> Subsystem1/3(end_time)
  phase time/1 -> Subsystem1/4(time)
  angular_vel/1 -> Subsystem1/6(angular_vel)
  angle_in/1 -> Subsystem1/5(current angle), Triggered Subsystem/1(angle_In)
  Subsystem1/1(torque) -> torque_out/1
  Triggered Subsystem/1(angle_Out) -> Subsystem1/1(initial angle)

== system pry_grasp_source/tentatively push/Enabled Subsystem2 ==
  In1 : Inport
  Enable : EnablePort
  Out1 : Outport  OutputWhenDisabled=reset  InitialOutput=0
  wires:
  In1/1 -> Out1/1

== system pry_grasp_source/tentatively push/Enabled Subsystem3 ==
  phase_start_time : Inport
  current_time : Inport  Port=2
  phase_end_time : Inport  Port=3
  Enable : EnablePort
  Relational Operator : RelationalOperator  OutDataTypeStr=boolean  RndMeth=Nearest
  Sum : Sum  Inputs=|-+
  phase_time : Outport  OutputWhenDisabled=reset  InitialOutput=0
  phase_end_signal : Outport  Port=2  OutputWhenDisabled=reset  InitialOutput=0
  wires:
  phase_start_time/1 -> Sum/1
  current_time/1 -> Sum/2
  Sum/1 -> phase_time/1, Relational Operator/1
  Relational Operator/1 -> phase_end_signal/1
  phase_end_time/1 -> Relational Operator/2

== system pry_grasp_source/tentatively push/Enabled Subsystem6 ==
  In1 : Inport
  Enable : EnablePort
  Out1 : Outport  OutputWhenDisabled=reset  InitialOutput=0
  wires:
  In1/1 -> Out1/1

== system pry_grasp_source/tentatively push/Triggered Subsystem1 ==
  Trigger : TriggerPort  VariantControl=(inherit)
  Constant : Constant  Value=[0 -2]
  Data Store Read : DataStoreRead  Priority=3  DataStoreName=phase_num
  Data Store Write : DataStoreWrite  DataStoreName=phase_num
  Sum : Sum  Inputs=|++
  wires:
  Data Store Read/1 -> Sum/1
  Sum/1 -> Data Store Write/1
  Constant/1 -> Sum/2

== system pry_grasp_source/tentatively push/Triggered Subsystem2 ==
  Trigger : TriggerPort  VariantControl=(inherit)
  Constant : Constant  Value=[0 1]
  Data Store Read : DataStoreRead  Priority=3  DataStoreName=phase_num
  Data Store Write : DataStoreWrite  DataStoreName=phase_num
  Sum : Sum  Inputs=|++
  wires:
  Data Store Read/1 -> Sum/1
  Sum/1 -> Data Store Write/1
  Constant/1 -> Sum/2

== system pry_grasp_source/tentatively push/Triggered Subsystem4 ==
  Trigger : TriggerPort  VariantControl=(inherit)
  Constant : Constant  Value=[0 -3]
  Data Store Read : DataStoreRead  Priority=3  DataStoreName=phase_num
  Data Store Write : DataStoreWrite  DataStoreName=phase_num
  Sum : Sum  Inputs=|++
  wires:
  Data Store Read/1 -> Sum/1
  Sum/1 -> Data Store Write/1
  Constant/1 -> Sum/2

== system pry_grasp_source/tentatively push/Triggered Subsystem5 ==
  In1 : Inport
  Trigger : TriggerPort  VariantControl=(inherit)
  Out1 : Outport  InitialOutput=0
  wires:
  In1/1 -> Out1/1

== system pry_grasp_source/phase1/Enabled Subsystem7/Subsystem ==
  initial_angle : Inport
  end_angle : Inport  Port=2
  end_time : Inport  Port=3
  time : Inport  Port=4
  angular_vel : Inport  Port=5
  current_angle : Inport  Port=6
  Enable : EnablePort
  Demux : Demux  Outputs=8
  Demux1 : Demux  Outputs=8
  MATLAB Function : MATLAB Function  TreatAsAtomicUnit=on
  Mux : Mux  Inputs=8
  PID1 : Subsystem
  PID2 : Subsystem
  PID3 : Subsystem
  PID4 : Subsystem
  PID5 : Subsystem
  PID6 : Subsystem
  PID7 : Subsystem
  PID8 : Subsystem
  Sum2 : Sum  Inputs=|+-
  torque_out : Outport  OutputWhenDisabled=reset  InitialOutput=[0 0 0 0 0 0 0 0]
  wires:
  initial_angle/1 -> MATLAB Function/1(initial_q)
  end_angle/1 -> MATLAB Function/2(end_q)
  time/1 -> MATLAB Function/4(time)
  end_time/1 -> MATLAB Function/3(end_time)
  angular_vel/1 -> Demux1/1
  MATLAB Function/1(angle_ref_out) -> Sum2/1
  Sum2/1 -> Demux/1
  current_angle/1 -> Sum2/2
  Mux/1 -> torque_out/1
  Demux/1 -> PID1/1(angle_error)
  Demux1/1 -> PID1/2(angular_vel)
  PID1/1(torque) -> Mux/1
  Demux/2 -> PID2/1(angle_error)
  Demux1/2 -> PID2/2(angular_vel)
  PID2/1(torque) -> Mux/2
  Demux/3 -> PID3/1(angle_error)
  Demux/4 -> PID4/1(angle_error)
  PID3/1(torque) -> Mux/3
  PID4/1(torque) -> Mux/4
  Demux/5 -> PID5/1(angle_error)
  PID5/1(torque) -> Mux/5
  PID6/1(torque) -> Mux/6
  Demux/6 -> PID6/1(angle_error)
  Demux1/3 -> PID3/2(angular_vel)
  Demux1/4 -> PID4/2(angular_vel)
  Demux1/5 -> PID5/2(angular_vel)
  Demux1/6 -> PID6/2(angular_vel)
  Demux/7 -> PID7/1(angle_error)
  Demux/8 -> PID8/1(angle_error)
  PID7/1(torque) -> Mux/7
  PID8/1(torque) -> Mux/8
  Demux1/7 -> PID7/2(angular_vel)
  Demux1/8 -> PID8/2(angular_vel)

== system pry_grasp_source/phase1/Enabled Subsystem7/Triggered Subsystem ==
  angle_In1 : Inport
  angle_ref_In2 : Inport  Port=2
  end_time_In3 : Inport  Port=3
  Trigger : TriggerPort  VariantControl=Variant
  angle_Out1 : Outport  InitialOutput=0
  angle_ref_Out2 : Outport  Port=2  InitialOutput=0
  end_time_Out3 : Outport  Port=3  InitialOutput=0
  wires:
  angle_In1/1 -> angle_Out1/1
  angle_ref_In2/1 -> angle_ref_Out2/1
  end_time_In3/1 -> end_time_Out3/1

== system pry_grasp_source/phase1-1/Enabled Subsystem7/Subsystem ==
  ref_angle : Inport
  angular_vel : Inport  Port=2
  current_angle : Inport  Port=3
  Enable : EnablePort
  Demux : Demux  Outputs=8
  Demux1 : Demux  Outputs=8
  Mux : Mux  Inputs=8
  PID1 : Subsystem
  PID2 : Subsystem
  PID3 : Subsystem
  PID4 : Subsystem
  PID5 : Subsystem
  PID6 : Subsystem
  PID7 : Subsystem
  PID8 : Subsystem
  Sum2 : Sum  Inputs=|+-
  torque_out : Outport  OutputWhenDisabled=reset  InitialOutput=[0 0 0 0 0 0 0 0]
  wires:
  angular_vel/1 -> Demux1/1
  ref_angle/1 -> Sum2/1
  Sum2/1 -> Demux/1
  current_angle/1 -> Sum2/2
  Mux/1 -> torque_out/1
  Demux/1 -> PID1/1(angle_error)
  Demux1/1 -> PID1/2(angular_vel)
  PID1/1(torque) -> Mux/1
  Demux/2 -> PID2/1(angle_error)
  Demux1/2 -> PID2/2(angular_vel)
  PID2/1(torque) -> Mux/2
  Demux/3 -> PID3/1(angle_error)
  Demux/4 -> PID4/1(angle_error)
  PID3/1(torque) -> Mux/3
  PID4/1(torque) -> Mux/4
  Demux/5 -> PID5/1(angle_error)
  PID5/1(torque) -> Mux/5
  PID6/1(torque) -> Mux/6
  Demux/6 -> PID6/1(angle_error)
  Demux1/3 -> PID3/2(angular_vel)
  Demux1/4 -> PID4/2(angular_vel)
  Demux1/5 -> PID5/2(angular_vel)
  Demux1/6 -> PID6/2(angular_vel)
  Demux/7 -> PID7/1(angle_error)
  Demux/8 -> PID8/1(angle_error)
  PID7/1(torque) -> Mux/7
  PID8/1(torque) -> Mux/8
  Demux1/7 -> PID7/2(angular_vel)
  Demux1/8 -> PID8/2(angular_vel)

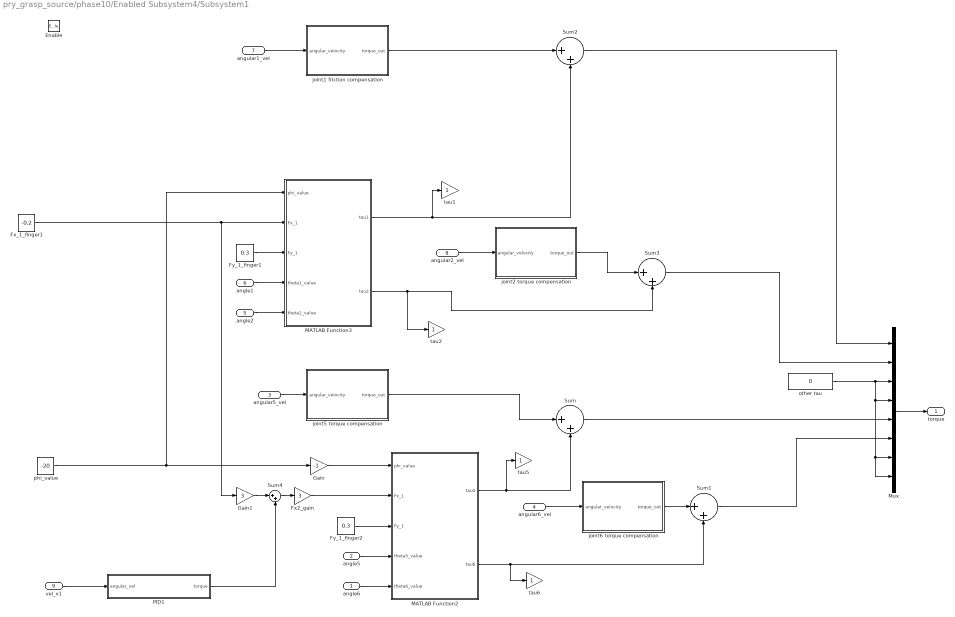
== system pry_grasp_source/phase10/Enabled Subsystem4/Subsystem1 ==
  angle6 : Inport
  angle5 : Inport  Port=2
  angular5_vel : Inport  Port=3
  angular6_vel : Inport  Port=4
  "angle2 " : Inport  Port=5
  angle1 : Inport  Port=6
  angular1_vel : Inport  Port=7
  angular2_vel : Inport  Port=8
  vel_x1 : Inport  Port=9
  Enable : EnablePort
  Fx2_gain : Gain  Gain=3
  Fx_1_finger1 : Constant  Value=-0.2
  Fy_1_finger1 : Constant  Value=0.3
  Fy_1_finger2 : Constant  Value=0.3
  Gain : Gain  Gain=-1
  Gain1 : Gain  Gain=3
  MATLAB Function2 : MATLAB Function  TreatAsAtomicUnit=on
  MATLAB Function3 : MATLAB Function  TreatAsAtomicUnit=on
  Mux : Mux  Inputs=8
  PID1 : Subsystem
  Sum{,1..4} (5 alike) : Sum  Inputs=|++
  joint1 friction compensation : Subsystem
  joint2 torque compensation : Subsystem
  joint5 torque compensation : Subsystem
  joint6 torque compensation : Subsystem
  other tau : Constant  Value=0
  phi_value : Constant  Value=-20
  tau{1..2,5..6} (4 alike) : Gain
  torque : Outport
  wires:
  Mux/1 -> torque/1
  other tau/1 -> Mux/8, Mux/7, Mux/4, Mux/3
  angle6/1 -> MATLAB Function2/5(theta6_value)
  Fy_1_finger2/1 -> MATLAB Function2/3(Fy_1)
  angle5/1 -> MATLAB Function2/4(theta5_value)
  Gain/1 -> MATLAB Function2/1(phi_value)
  angular5_vel/1 -> joint5 torque compensation/1(angular_velocity)
  MATLAB Function2/1(tau5) -> tau5/1, Sum/2
  joint5 torque compensation/1(torque_out) -> Sum/1
  angular6_vel/1 -> joint6 torque compensation/1(angular_velocity)
  joint6 torque compensation/1(torque_out) -> Sum1/1
  MATLAB Function2/2(tau6) -> tau6/1, Sum1/2
  Fx_1_finger1/1 -> Gain1/1, MATLAB Function3/2(Fx_1)
  Fy_1_finger1/1 -> MATLAB Function3/3(Fy_1)
  phi_value/1 -> MATLAB Function3/1(phi_value), Gain/1
  angle1/1 -> MATLAB Function3/4(theta1_value)
  "angle2 "/1 -> MATLAB Function3/5(theta2_value)
  joint1 friction compensation/1(torque_out) -> Sum2/1
  angular1_vel/1 -> joint1 friction compensation/1(angular_velocity)
  MATLAB Function3/1(tau1) -> tau1/1, Sum2/2
  joint2 torque compensation/1(torque_out) -> Sum3/1
  MATLAB Function3/2(tau2) -> tau2/1, Sum3/2
  angular2_vel/1 -> joint2 torque compensation/1(angular_velocity)
  Sum3/1 -> Mux/2
  Sum2/1 -> Mux/1
  Sum/1 -> Mux/5
  Sum1/1 -> Mux/6
  Gain1/1 -> Sum4/1
  vel_x1/1 -> PID1/1(angular_vel)
  PID1/1(torque) -> Sum4/2
  Sum4/1 -> Fx2_gain/1
  Fx2_gain/1 -> MATLAB Function2/2(Fx_1)

== system pry_grasp_source/phase11/Enabled Subsystem4/Subsystem1 ==
  "angle2 " : Inport
  angle1 : Inport  Port=2
  angle6 : Inport  Port=3
  angle5 : Inport  Port=4
  Enable : EnablePort
  Fx_1_finger1 : Constant
  Fy_1_finger1 : Constant  Value=0.1
  Fy_1_finger2 : Constant  Value=0.1
  Gain : Gain  Gain=-1
  MATLAB Function1 : MATLAB Function  TreatAsAtomicUnit=on
  MATLAB Function2 : MATLAB Function  TreatAsAtomicUnit=on
  Mux : Mux  Inputs=8
  offset : Gain  Gain=0.3
  other tau : Constant  Value=0
  phi_value : Constant  Value=-16
  torque : Outport
  wires:
  Mux/1 -> torque/1
  other tau/1 -> Mux/8, Mux/7, Mux/4, Mux/3
  MATLAB Function1/2(tau2) -> Mux/2
  angle1/1 -> MATLAB Function1/4(theta1_value)
  phi_value/1 -> Gain/1, MATLAB Function1/1(phi_value)
  MATLAB Function1/1(tau1) -> Mux/1
  Fy_1_finger1/1 -> MATLAB Function1/3(Fy_1)
  "angle2 "/1 -> MATLAB Function1/5(theta2_value)
  Fx_1_finger1/1 -> offset/1, MATLAB Function1/2(Fx_1)
  angle6/1 -> MATLAB Function2/5(theta6_value)
  Fy_1_finger2/1 -> MATLAB Function2/3(Fy_1)
  angle5/1 -> MATLAB Function2/4(theta5_value)
  offset/1 -> MATLAB Function2/2(Fx_1)
  MATLAB Function2/1(tau5) -> Mux/5
  MATLAB Function2/2(tau6) -> Mux/6
  Gain/1 -> MATLAB Function2/1(phi_value)

== system pry_grasp_source/phase2/Enabled Subsystem7/Subsystem ==
  ref_angle : Inport
  angular_vel : Inport  Port=2
  current_angle : Inport  Port=3
  Enable : EnablePort
  Demux : Demux  Outputs=8
  Demux1 : Demux  Outputs=8
  Mux : Mux  Inputs=8
  PID1 : Subsystem
  PID2 : Subsystem
  PID3 : Subsystem
  PID4 : Subsystem
  PID5 : Subsystem
  PID6 : Subsystem
  PID7 : Subsystem
  PID8 : Subsystem
  Sum2 : Sum  Inputs=|+-
  torque_out : Outport  OutputWhenDisabled=reset  InitialOutput=[0 0 0 0 0 0 0 0]
  wires:
  angular_vel/1 -> Demux1/1
  ref_angle/1 -> Sum2/1
  Sum2/1 -> Demux/1
  current_angle/1 -> Sum2/2
  Mux/1 -> torque_out/1
  Demux/1 -> PID1/1(angle_error)
  Demux1/1 -> PID1/2(angular_vel)
  PID1/1(torque) -> Mux/1
  Demux/2 -> PID2/1(angle_error)
  Demux1/2 -> PID2/2(angular_vel)
  PID2/1(torque) -> Mux/2
  Demux/3 -> PID3/1(angle_error)
  Demux/4 -> PID4/1(angle_error)
  PID3/1(torque) -> Mux/3
  PID4/1(torque) -> Mux/4
  Demux/5 -> PID5/1(angle_error)
  PID5/1(torque) -> Mux/5
  PID6/1(torque) -> Mux/6
  Demux/6 -> PID6/1(angle_error)
  Demux1/3 -> PID3/2(angular_vel)
  Demux1/4 -> PID4/2(angular_vel)
  Demux1/5 -> PID5/2(angular_vel)
  Demux1/6 -> PID6/2(angular_vel)
  Demux/7 -> PID7/1(angle_error)
  Demux/8 -> PID8/1(angle_error)
  PID7/1(torque) -> Mux/7
  PID8/1(torque) -> Mux/8
  Demux1/7 -> PID7/2(angular_vel)
  Demux1/8 -> PID8/2(angular_vel)

== system pry_grasp_source/phase6.1/Enabled Subsystem7/Subsystem ==
  initial_angle : Inport
  end_angle : Inport  Port=2
  end_time : Inport  Port=3
  time : Inport  Port=4
  angular_vel : Inport  Port=5
  current_angle : Inport  Port=6
  Enable : EnablePort
  Demux : Demux  Outputs=8
  Demux1 : Demux  Outputs=8
  MATLAB Function : MATLAB Function  TreatAsAtomicUnit=on
  Mux : Mux  Inputs=8
  PID1 : Subsystem
  PID2 : Subsystem
  PID3 : Subsystem
  PID4 : Subsystem
  PID5 : Subsystem
  PID6 : Subsystem
  PID7 : Subsystem
  PID8 : Subsystem
  Sum2 : Sum  Inputs=|+-
  angle error : Gain
  tau1 : Gain
  tau_out : Outport
  wires:
  initial_angle/1 -> MATLAB Function/1(initial_q)
  end_angle/1 -> MATLAB Function/2(end_q)
  time/1 -> MATLAB Function/4(time)
  end_time/1 -> MATLAB Function/3(end_time)
  angular_vel/1 -> Demux1/1
  MATLAB Function/1(angle_ref_out) -> Sum2/1
  Sum2/1 -> angle error/1, Demux/1
  current_angle/1 -> Sum2/2
  Mux/1 -> tau_out/1
  Demux/1 -> PID1/1(angle_error)
  Demux1/1 -> PID1/2(angular_vel)
  PID1/1(torque) -> tau1/1, Mux/1
  Demux/2 -> PID2/1(angle_error)
  Demux1/2 -> PID2/2(angular_vel)
  PID2/1(torque) -> Mux/2
  Demux/3 -> PID3/1(angle_error)
  Demux/4 -> PID4/1(angle_error)
  PID3/1(torque) -> Mux/3
  PID4/1(torque) -> Mux/4
  Demux/5 -> PID5/1(angle_error)
  PID5/1(torque) -> Mux/5
  PID6/1(torque) -> Mux/6
  Demux/6 -> PID6/1(angle_error)
  Demux1/3 -> PID3/2(angular_vel)
  Demux1/4 -> PID4/2(angular_vel)
  Demux1/5 -> PID5/2(angular_vel)
  Demux1/6 -> PID6/2(angular_vel)
  Demux/7 -> PID7/1(angle_error)
  Demux/8 -> PID8/1(angle_error)
  PID7/1(torque) -> Mux/7
  PID8/1(torque) -> Mux/8
  Demux1/7 -> PID7/2(angular_vel)
  Demux1/8 -> PID8/2(angular_vel)

== system pry_grasp_source/phase6.1/Enabled Subsystem7/Triggered Subsystem ==
  angle_In1 : Inport
  angle_ref_In2 : Inport  Port=2
  end_time_In3 : Inport  Port=3
  Trigger : TriggerPort  VariantControl=Variant
  angle_Out1 : Outport  InitialOutput=0
  angle_ref_Out2 : Outport  Port=2  InitialOutput=0
  end_time_Out3 : Outport  Port=3  InitialOutput=0
  wires:
  angle_In1/1 -> angle_Out1/1
  angle_ref_In2/1 -> angle_ref_Out2/1
  end_time_In3/1 -> end_time_Out3/1
